simulink model "rahul_loaded"  (R2015a)
settings: Solver=ode45  StartTime=0.0  StopTime=20  RelTol=1e-3
undefined symbols (not defined in the file): sigbuilder_block
settings Model: Creator=Nitesh  LastModifiedBy=Nitesh
settings DataIOCC: LimitDataPoints=off

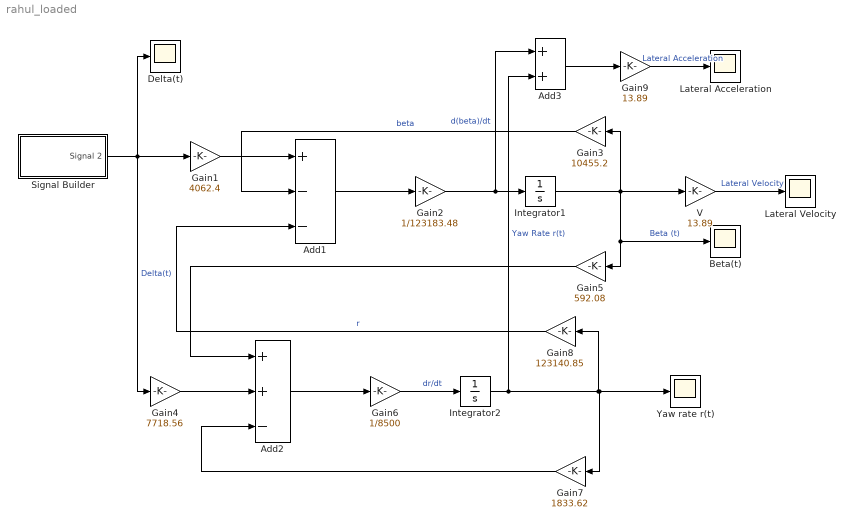
== system rahul_loaded ==
  Add1 : Sum  Inputs=+--
  Add2 : Sum  Inputs=++-
  Add3 : Sum
  Beta(t) : Scope
      settings: SaveName=ScopeData2
  Delta(t) : Scope
  Gain1 : Gain  Gain=4062.4
  Gain2 : Gain  Gain=1/123183.48
  Gain3 : Gain  Gain=10455.2
  Gain4 : Gain  Gain=7718.56
  Gain5 : Gain  Gain=592.08
  Gain6 : Gain  Gain=1/8500
  Gain7 : Gain  Gain=1833.62
  Gain8 : Gain  Gain=123140.85
  Gain9 : Gain  Gain=13.89
  Integrator1 : Integrator
  Integrator2 : Integrator
  Lateral Acceleration : Scope
      settings: SaveName=ScopeData4
  Lateral Velocity : Scope
      settings: SaveName=ScopeData3
  Signal Builder : Subsystem  Tag=STV Subsys  LoadFcn=sigbuilder_block('load');  StartFcn=sigbuilder_block('start');  StopFcn=sigbuilder_block('stop');  ClipboardFcn=sigbuilder_block('clipboard');  mask(Sigbuilder block){}
      mask help: Simulink:masks:SigbuilderBlock_MD
      mask init:
      | if ~strcmp(get_param(bdroot(gcbh),'SimulationStatus'),'stopped') tuvar = sigbuilder_block('maskInit'); end
      settings: CopyFcn=sigbuilder_block('copy');  DeleteFcn=sigbuilder_block('delete');  ModelCloseFcn=sigbuilder_block('modelClose');  PreSaveFcn=sigbuilder_block('preSave');  PauseFcn=sigbuilder_block('pause');  ContinueFcn=sigbuilder_block('continue');  NameChangeFcn=sigbuilder_block('namechange');  OpenFcn=sigbuilder_block('open',[437.6 199.2 550.4 400 ]);  CloseFcn=sigbuilder_block('close');
      mask Display: plot(0, 0, 100, 100,[2, 2, 32, 32, 2], [68, 8, 8, 68, 68],[32, 2], [38, 38], [32, 19, 2],[53, 60, 44], [32, 17, 17, 2],[16, 16, 31, 31]);txt = getActiveGroup(gcbh);text(2, 100, txt,'verticalAlignment', 'top');
  V : Gain  Gain=13.89
  Yaw rate r(t) : Scope
  wires:
  Signal Builder/1(Signal 2) -> Delta(t)/1, Gain4/1, Gain1/1  "Delta(t)"
  Gain1/1 -> Add1/1
  Gain3/1 -> Add1/2  "beta"
  Gain8/1 -> Add1/3  "r"
  Add1/1 -> Gain2/1
  Gain2/1 -> Add3/1, Integrator1/1  "d(beta)/dt"
  Integrator1/1 -> V/1, Beta(t)/1, Gain5/1, Gain3/1  "Beta (t)"
  Gain4/1 -> Add2/2
  Gain5/1 -> Add2/1
  Add2/1 -> Gain6/1
  Gain6/1 -> Integrator2/1  "dr/dt"
  Integrator2/1 -> Yaw rate r(t)/1, Gain7/1, Gain8/1, Add3/2  "Yaw Rate r(t)"
  Gain7/1 -> Add2/3
  V/1 -> Lateral Velocity/1  "Lateral Velocity"
  Add3/1 -> Gain9/1
  Gain9/1 -> Lateral Acceleration/1  "Lateral Acceleration"

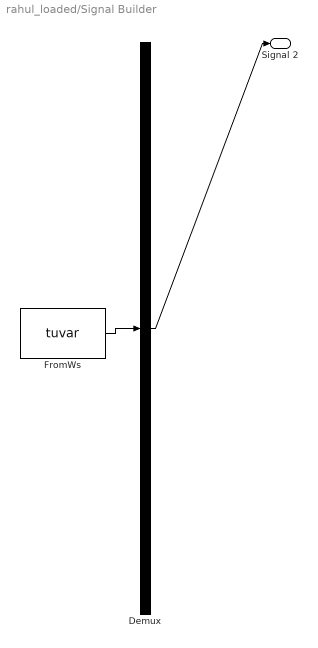
== system rahul_loaded/Signal Builder ==
  Demux : Demux  Tag=STV Demux  Outputs=1
  FromWs : FromWorkspace  Tag=STV FromWs  VariableName=tuvar  SampleTime=0
      SigBuilderData=|
      | common.afterFinalStr = 'Extrapolate'
      | common.sampleTime = 0
      | dataSet.timeRange = [0 8]
      | dataSet.name = 'Group 1'
      | sbobj.Groups.Name = 'Group 1'
      | sbobj.Groups.Signals.Name = 'Signal 2'
      | sbobj.Groups.Signals.XData = [0 0.5 8]
      | sbobj.Groups.Signals.YData = [0 2 2]
      | sbobj.Groups.TimeRange = [0 8]
  Signal 2 : Outport  Tag=STV Outport
  wires:
  FromWs/1 -> Demux/1
  Demux/1 -> Signal 2/1
